simulink model "PerturbedCartesianOrbitPropagator"  (R2023a)
settings: Solver=ode4  StartTime=0.0  StopTime=10.0  FixedStep=dt  MaxStep=max_step_size  RelTol=relative_tolerance
undefined symbols (not defined in the file or in its folder): J2_flag, srp_flag, sun_grav_flag
settings Model: Creator=ndelurgio  LastModifiedBy=ndelurgio

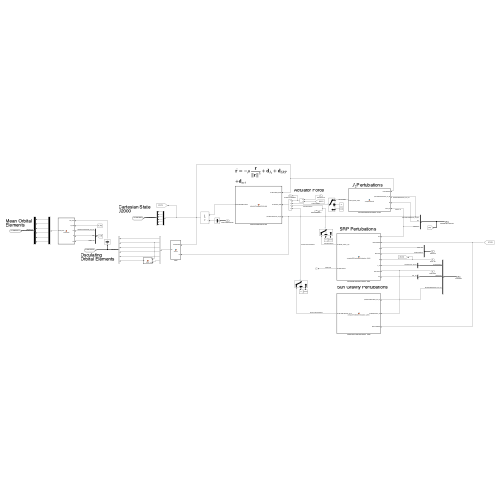
[thumbnail: Simulink's stored preview of the top-level diagram]
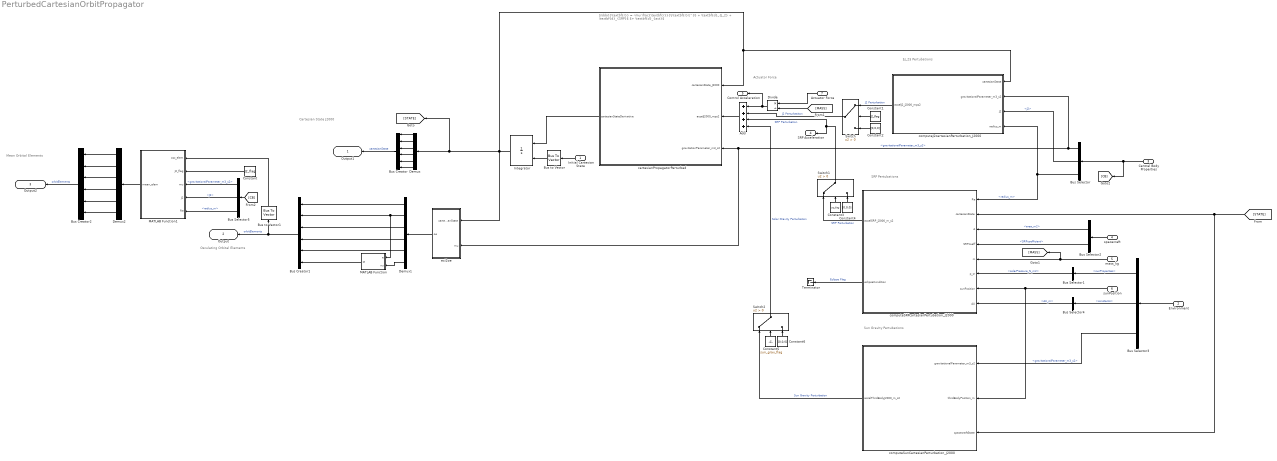
== system PerturbedCartesianOrbitPropagator ==
  note: $J_2$ Pertubations
  note: $\ddot{\textbf{r}} = -\mu \frac{\textbf{r}}{\|\textbf{r}\|^3} + \textbf{d}_{J_2} + \textbf{d}_{SRP}$ $+ \textbf{d}_{act}$
  note: SRP Pertubations
  note: Actuator Force
  note: Cartesian State J2000
  note: Mean Orbital Elements
  note: Osculating Orbital Elements
  note: Sun Gravity Pertubations
  Initial Cartesian State : Inport  OutDataTypeStr=Bus: cartesianState
  Environment : Inport  Port=2  OutDataTypeStr=Bus: environmentBus
  Central Body Properties : Inport  Port=3  OutDataTypeStr=Bus: planetProperties
  spacecraft : Inport  Port=4  OutDataTypeStr=Bus: properties
  mass_kg : Inport  Port=5
  sunPosition : Inport  Port=6  PortDimensions=3
  Actuator Force : Inport  Port=7  PortDimensions=3
  Add : Sum  Inputs=++++
  Bus Creator : BusCreator  Inputs=6  OutDataTypeStr=Bus: cartesianState  NonVirtualBus=on
      settings: InheritFromInputs=off
  Bus Creator1 : BusCreator  Inputs=6  OutDataTypeStr=Bus: osculatingOrbitElements
      settings: InheritFromInputs=off
  Bus Creator2 : BusCreator  Inputs=6  OutDataTypeStr=Bus: osculatingOrbitElements  NonVirtualBus=on
      settings: InheritFromInputs=off
  Bus Selector : BusSelector  OutputSignals=gravitationalParameter_m3_s2,J2,radius_m
  Bus Selector1 : BusSelector  OutputSignals=solarPressure_N_m2
  Bus Selector2 : BusSelector  OutputSignals=area_m2,SRPcoefficient
  Bus Selector3 : BusSelector  OutputSignals=sunProperties,constants,sunProperties.gravitationalParameter_m3_s2
  Bus Selector4 : BusSelector  OutputSignals=AU_m
  Bus Selector5 : BusSelector  OutputSignals=gravitationalParameter_m3_s2,J2,radius_m
  Bus to Vector : BusToVector
  Bus to Vector1 : BusToVector
  Constant : Constant  Value=J2_flag
  Constant1 : Constant  Value=J2_flag
  Constant2 : Constant  Value=[0,0,0]
  Constant3 : Constant  Value=srp_flag
  Constant4 : Constant  Value=[0,0,0]
  Constant5 : Constant  Value=sun_grav_flag
  Constant6 : Constant  Value=[0,0,0]
  Demux : Demux  Outputs=6
  Demux1 : Demux  Outputs=6
  Demux2 : Demux  Outputs=6
  Divide : Product  Inputs=*/
  Integrator : Integrator  InitialConditionSource=external
  MATLAB Function : MATLAB Function  TreatAsAtomicUnit=on
  MATLAB Function1 : MATLAB Function  TreatAsAtomicUnit=on
  Switch : Switch  Criteria=u2 > Threshold  SaturateOnIntegerOverflow=off  InputSameDT=off
  Switch1 : Switch  Criteria=u2 > Threshold  SaturateOnIntegerOverflow=off  InputSameDT=off
  Switch2 : Switch  Criteria=u2 > Threshold  SaturateOnIntegerOverflow=off  InputSameDT=off
  Terminator : Terminator
  cartesianPropagatorPerturbed : MATLAB Function  TreatAsAtomicUnit=on
  computeJ2cartesianPerturbation_J2000 : MATLAB Function  TreatAsAtomicUnit=on
  computeSRPcartesianPertubation_J2000 : MATLAB Function  TreatAsAtomicUnit=on
  computeSunCartesianPerturbation_J2000 : MATLAB Function  TreatAsAtomicUnit=on
  eci2oe : MATLAB Function  TreatAsAtomicUnit=on
  Output1 : Outport  OutDataTypeStr=Bus: cartesianState
  Output : Outport  Port=2  OutDataTypeStr=Bus: osculatingOrbitElements
  Output2 : Outport  Port=3  OutDataTypeStr=Bus: meanOrbitElements
  SRP Acceleration : Outport  Port=4
  Control Acceleration : Outport  Port=5
  wires:
  computeJ2cartesianPerturbation_J2000/1(accelJ2_J2000_mps2) -> Switch/1  "J2 Perturbation"
  Environment/1 -> Bus Selector3/1
  Bus Selector/2 -> computeJ2cartesianPerturbation_J2000/3(J2)  "<J2>"
  Demux/2 -> Bus Creator/2
  Bus Creator/1 -> Output1/1  "cartesianState"
  Demux/3 -> Bus Creator/3
  Demux/1 -> Bus Creator/1
  Demux/6 -> Bus Creator/6
  Demux/5 -> Bus Creator/5
  Demux/4 -> Bus Creator/4
  Bus to Vector/1 -> Integrator/2
  cartesianPropagatorPerturbed/1(cartesianStateDerivative) -> Integrator/1
  Initial Cartesian State/1 -> Bus to Vector/1
  Integrator/1 -> [STATE], Demux/1, eci2oe/1(cartesianState), computeJ2cartesianPerturbation_J2000/1(cartesianState), cartesianPropagatorPerturbed/1(cartesianState_J2000)
  Demux1/6 -> MATLAB Function/2(nu)
  Demux1/4 -> Bus Creator1/4
  Demux1/5 -> Bus Creator1/5
  Bus Creator1/1 -> Bus to Vector1/1, Output/1  "orbitElements"
  Demux1/3 -> Bus Creator1/3
  Demux1/2 -> MATLAB Function/1(e), Bus Creator1/2
  Demux1/1 -> Bus Creator1/1
  MATLAB Function/1(M) -> Bus Creator1/6
  Bus to Vector1/1 -> MATLAB Function1/1(osc_elem)
  Constant/1 -> MATLAB Function1/2(J2_flag)
  MATLAB Function1/1(mean_elem) -> Demux2/1
  Demux2/4 -> Bus Creator2/4
  Demux2/3 -> Bus Creator2/3
  Demux2/5 -> Bus Creator2/5
  Demux2/2 -> Bus Creator2/2
  Demux2/1 -> Bus Creator2/1
  Demux2/6 -> Bus Creator2/6
  Bus Creator2/1 -> Output2/1  "orbitElements"
  Switch/1 -> Add/2  "J2 Perturbtaiton"
  Constant1/1 -> Switch/2
  Constant2/1 -> Switch/3
  Bus Selector/1 -> eci2oe/2(mu), cartesianPropagatorPerturbed/3(gravitationParameter_m3_s2), computeJ2cartesianPerturbation_J2000/2(gravitationalParameter_m3_s2)  "<gravitationalParameter_m3_s2>"
  Bus Selector/3 -> computeJ2cartesianPerturbation_J2000/4(radius_m), computeSRPcartesianPertubation_J2000/1(Re)  "<radius_m>"
  Bus Selector1/1 -> computeSRPcartesianPertubation_J2000/6(p_sr)  "<solarPressure_N_m2>"
  [STATE] -> computeSunCartesianPerturbation_J2000/3(spacecraftState), computeSRPcartesianPertubation_J2000/2(cartesianState)
  computeSRPcartesianPertubation_J2000/1(accelSRP_J2000_m_s2) -> Switch1/1  "SRP Perturbation"
  spacecraft/1 -> Bus Selector2/1
  sunPosition/1 -> computeSunCartesianPerturbation_J2000/2(thirdBodyPosition_m), computeSRPcartesianPertubation_J2000/7(sunPosition)
  Bus Selector2/1 -> computeSRPcartesianPertubation_J2000/3(A)  "<area_m2>"
  Bus Selector2/2 -> computeSRPcartesianPertubation_J2000/4(SRPcoeff)  "<SRPcoefficient>"
  mass_kg/1 -> [MASS], computeSRPcartesianPertubation_J2000/5(m)
  computeSRPcartesianPertubation_J2000/2(eclipseCondition) -> Terminator/1  "Eclipse Flag"
  Bus Selector3/1 -> Bus Selector1/1  "<sunProperties>"
  Bus Selector3/2 -> Bus Selector4/1  "<constants>"
  Bus Selector4/1 -> computeSRPcartesianPertubation_J2000/8(AU)  "<AU_m>"
  Constant3/1 -> Switch1/2
  Constant4/1 -> Switch1/3
  Switch1/1 -> Add/3, SRP Acceleration/1  "SRP Perturbation"
  Add/1 -> cartesianPropagatorPerturbed/2(accelJ2000_mps2)
  Actuator Force/1 -> Divide/1
  Divide/1 -> Add/1, Control Acceleration/1
  [MASS] -> Divide/2
  Central Body Properties/1 -> [CB], Bus Selector/1
  [CB] -> Bus Selector5/1
  Bus Selector5/2 -> MATLAB Function1/4(J2)  "<J2>"
  Bus Selector5/1 -> MATLAB Function1/3(mu)  "<gravitationalParameter_m3_s2>"
  Bus Selector5/3 -> MATLAB Function1/5(Re)  "<radius_m>"
  eci2oe/1(oe) -> Demux1/1
  Bus Selector3/3 -> computeSunCartesianPerturbation_J2000/1(gravitationalParameter_m3_s2)  "<gravitationalParameter_m3_s2>"
  Constant6/1 -> Switch2/3
  Constant5/1 -> Switch2/2
  computeSunCartesianPerturbation_J2000/1(accelThirdBodyJ2000_m_s2) -> Switch2/1  "Sun Gravity Perturbation"
  Switch2/1 -> Add/4  "Solar Gravity Perturbation"

== matlab function PerturbedCartesianOrbitPropagator/cartesianPropagatorPerturbed ==
  data: cartesianState_J2000 input; cartesianStateDerivative output; accelJ2000_mps2 input; gravitationParameter_m3_s2 input
function cartesianStateDerivative = cartesianPropagatorPerturbed(cartesianState_J2000,accelJ2000_mps2,gravitationParameter_m3_s2)

cartesianStateDerivative = cartesianPropagatorPerturbed(cartesianState_J2000,accelJ2000_mps2,gravitationParameter_m3_s2);

end

== matlab function PerturbedCartesianOrbitPropagator/computeJ2cartesianPerturbation_J2000 ==
  data: cartesianState input; accelJ2_J2000_mps2 output; gravitationalParameter_m3_s2 input; J2 input; radius_m input
function accelJ2_J2000_mps2 = computeJ2accel(cartesianState,gravitationalParameter_m3_s2,J2,radius_m)

accelJ2_J2000_mps2 = computeJ2cartesianPerturbation_J2000(cartesianState,gravitationalParameter_m3_s2,J2,radius_m);

end

== matlab function PerturbedCartesianOrbitPropagator/eci2oe ==
  data: cartesianState input; oe output; mu input
function oe = eci2oe(cartesianState,mu)
[oe,~,~,~] = eci2oe( cartesianState , mu );
end

== matlab function PerturbedCartesianOrbitPropagator/MATLAB Function ==
  data: e input; M output; nu input
function M = nu2M(e,nu)
M = nu2M(nu,e);
end

== matlab function PerturbedCartesianOrbitPropagator/MATLAB Function1 ==
  data: osc_elem input; mean_elem output; J2_flag input; mu input; J2 input; Re input
function mean_elem = osc2mean(osc_elem, J2_flag, mu, J2, Re)
mean_elem = osc2mean(osc_elem, J2_flag, mu, J2, Re);
end

== matlab function PerturbedCartesianOrbitPropagator/computeSRPcartesianPertubation_J2000 ==
  data: Re input; cartesianState input; accelSRP_J2000_m_s2 output; A input; SRPcoeff input; m input; p_sr input; sunPosition input; eclipseCondition output; AU input
function [accelSRP_J2000_m_s2, eclipseCondition] = computeSRPcartesianPertubation_J2000(Re, cartesianState, A, SRPcoeff, m, p_sr, sunPosition, AU)

[accelSRP_J2000_m_s2, eclipseCondition] = computeSRPcartesianPertubation_J2000(cartesianState, A, SRPcoeff, m, p_sr, sunPosition, Re, AU);

end

== matlab function PerturbedCartesianOrbitPropagator/computeSunCartesianPerturbation_J2000 ==
  data: gravitationalParameter_m3_s2 input; accelThirdBodyJ2000_m_s2 output; thirdBodyPosition_m input; spacecraftState input
function accelThirdBodyJ2000_m_s2 = computeThirdBodyPerturbation_J2000(gravitationalParameter_m3_s2,thirdBodyPosition_m,spacecraftState)
accelThirdBodyJ2000_m_s2 = computeThirdBodyPerturbation_J2000(gravitationalParameter_m3_s2,thirdBodyPosition_m,spacecraftState);
end
